simulink model "bloque1a"  (Simulink 5.0)
settings: Solver=ode45  StartTime=0.0  StopTime=75.0  RelTol=1e-3
undefined symbols (not defined in the file): q, Vd, Vm
settings Model: LastModifiedBy=pc1

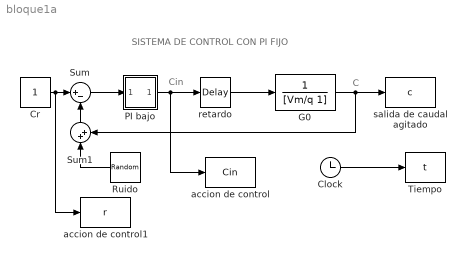
== system bloque1a ==
  note: Cin
  note: C
  note: SISTEMA DE CONTROL CON PI FIJO
  Clock : Clock
      settings: Decimation=10
  Cr : Constant
  G0 : TransferFcn  Denominator=[Vm/q 1]
  PI bajo : Subsystem  AncestorBlock=simulink_extras/Additional Linear/PID Controller  mask(PID Controller){P=0.9, I=0.9/1.578, D=0}
      mask prompts: P "Proportional:"; I "Integral:"; D "Derivative:"
      mask help:
      | Enter expressions for proportional, integral, and derivative terms.
      | P+I/s+Ds
      mask Help: This block implements a PID controller where parameters are entered for the Proportional, Integral and Derivative terms. Unmask this block to see how it works. The derivative term is implemented using a true derivative block.
      mask Display: disp('PID')
  Ruido : RandomNumber  Orientation=left  Variance=0.01  Seed=5  SampleTime=0.1
  Sum : Sum  Inputs=|+-  SaturateOnIntegerOverflow=on
  Sum1 : Sum  Orientation=up  Inputs=|++  SaturateOnIntegerOverflow=on
  Tiempo : ToWorkspace  VariableName=t  SampleTime=-1  SaveFormat=Array
  accion de control : ToWorkspace  VariableName=Cin  SampleTime=-1  SaveFormat=Array
  accion de control1 : ToWorkspace  VariableName=r  SampleTime=-1  SaveFormat=Array
  retardo : TransportDelay  DelayTime=Vd/q
  salida de caudal agitado : ToWorkspace  VariableName=c  SampleTime=-1  SaveFormat=Array
  wires:
  Cr/1 -> Sum/1, accion de control1/1
  Sum/1 -> PI bajo/1(In)
  PI bajo/1(Out) -> retardo/1, accion de control/1
  retardo/1 -> G0/1
  G0/1 -> salida de caudal agitado/1, Sum1/2
  Clock/1 -> Tiempo/1
  Sum1/1 -> Sum/2
  Ruido/1 -> Sum1/1

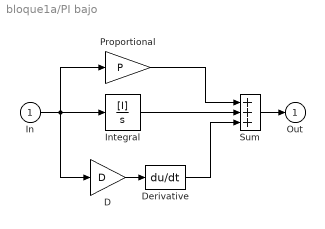
== system bloque1a/PI bajo ==
  In : Inport
  D : Gain  Gain=D  SaturateOnIntegerOverflow=on
  Derivative : Derivative
  Integral : TransferFcn  Numerator=[I]  Denominator=[1 0]
  Proportional : Gain  Gain=P  SaturateOnIntegerOverflow=on
  Sum : Sum  Inputs=+++  SaturateOnIntegerOverflow=on  InputSameDT=on
  Out : Outport  InitialOutput=0
  wires:
  Proportional/1 -> Sum/1
  Integral/1 -> Sum/2
  Derivative/1 -> Sum/3
  In/1 -> Integral/1, Proportional/1, D/1
  Sum/1 -> Out/1
  D/1 -> Derivative/1
